simulink model "CM670A_HwAg1Meas"  (R2013b)
settings: Solver=FixedStepDiscrete  SolverMode=SingleTasking  StartTime=0.0  StopTime=22  FixedStep=0.002  RelTol=1e-3
values from neighbouring files (symbols this model uses):
  ELECGLBPRM_DEGPERREV_DEGPERREV_F32 = DataDict.Constant    [CM670A_HwAg1Meas_DataDict.m]
  ELECGLBPRM_HWAGCENTROFFS_HWDEG_F32 = DataDict.Constant    [CM670A_HwAg1Meas_DataDict.m]
  ELECGLBPRM_HWAGSATNLOWRLIM_HWDEG_F32 = DataDict.Constant    [CM670A_HwAg1Meas_DataDict.m]
  ELECGLBPRM_HWAGSATNUPPRLIM_HWDEG_F32 = DataDict.Constant    [CM670A_HwAg1Meas_DataDict.m]
  ELECGLBPRM_HWAGSCA_ULS_F32 = DataDict.Constant    [CM670A_HwAg1Meas_DataDict.m]
  ELECGLBPRM_HWAGSPURGEARRAT_ULS_F32 = DataDict.Constant    [CM670A_HwAg1Meas_DataDict.m]
  ELECGLBPRM_HWAGSPURTORINGGEARRATSNSR0_ULS_F32 = DataDict.Constant    [CM670A_HwAg1Meas_DataDict.m]
  ELECGLBPRM_HWAGSPURTORINGGEARRATSNSR1_ULS_F32 = DataDict.Constant    [CM670A_HwAg1Meas_DataDict.m]
  ELECGLBPRM_NOFLT_CNT_U08 = DataDict.Constant    [CM670A_HwAg1Meas_DataDict.m]
  ELECGLBPRM_OFFSTRIMNOTPRFMD_CNT_U08 = DataDict.Constant    [CM670A_HwAg1Meas_DataDict.m]
  ELECGLBPRM_PRTCLFLT_CNT_U08 = DataDict.Constant    [CM670A_HwAg1Meas_DataDict.m]
  ELECGLBPRM_SKIPSTEPFLT_CNT_U08 = DataDict.Constant    [CM670A_HwAg1Meas_DataDict.m]
  ELECGLBPRM_SNSRINTFLT_CNT_U08 = DataDict.Constant    [CM670A_HwAg1Meas_DataDict.m]
  ELECGLBPRM_VRNRERRFLT_CNT_U08 = DataDict.Constant    [CM670A_HwAg1Meas_DataDict.m]
  HWAG10THTOOTHTRIG_CNT_U08 = DataDict.ConfigParam    [CM670A_HwAg1Meas_DataDict.m]
  HWAG11THTOOTHTRIG_CNT_U08 = DataDict.ConfigParam    [CM670A_HwAg1Meas_DataDict.m]
  HwAg1IfFlt = DataDict.NTC    [CM670A_HwAg1Meas_DataDict.m]
  HwAg1MeasHwAg1IfFltFailStep = DataDict.Calibration    [CM670A_HwAg1Meas_DataDict.m]
  HwAg1MeasHwAg1IfFltPassStep = DataDict.Calibration    [CM670A_HwAg1Meas_DataDict.m]
  HwAg1MeasHwAg1Snsr0PrtclFltFailStep = DataDict.Calibration    [CM670A_HwAg1Meas_DataDict.m]
  HwAg1MeasHwAg1Snsr0PrtclFltPassStep = DataDict.Calibration    [CM670A_HwAg1Meas_DataDict.m]
  HwAg1MeasHwAg1Snsr1PrtclFltFailStep = DataDict.Calibration    [CM670A_HwAg1Meas_DataDict.m]
  HwAg1MeasHwAg1Snsr1PrtclFltPassStep = DataDict.Calibration    [CM670A_HwAg1Meas_DataDict.m]
  HwAg1MeasSnsr0Rev = DataDict.Calibration    [CM670A_HwAg1Meas_DataDict.m]
  HwAg1MeasSnsr1Rev = DataDict.Calibration    [CM670A_HwAg1Meas_DataDict.m]
  HwAg1MeasStep = DataDict.Calibration    [CM670A_HwAg1Meas_DataDict.m]
  HwAg1MeasVrnrErrThd = DataDict.Calibration    [CM670A_HwAg1Meas_DataDict.m]
  HwAg1MfgFlt = DataDict.NTC    [CM670A_HwAg1Meas_DataDict.m]
  HwAg1Snsr0PrtclFlt = DataDict.NTC    [CM670A_HwAg1Meas_DataDict.m]
  HwAg1Snsr1PrtclFlt = DataDict.NTC    [CM670A_HwAg1Meas_DataDict.m]
undefined symbols (not defined in the file or in its folder): NtcSts1, sigbuilder_block, SigQlfr1
libraries: simulink x30, NxtrNvM x3
(part 2 of 5)

== system CM670A_HwAg1Meas/HwAg1Meas/HwAg1MeasPer3 ==
  note: Follow below steps in same order:
      |
      | 1. Check the Sensor Seq Number
      |    1a. Check Sensor Seq Number Logic first
      |    1b. Execute RawHwAgRead
      |    1c. Clear RSENT2CSC = 2046U;
      |    1d. FRS Flag Check: If the RegInpRSENT2FRS==1,  Read the RegInpRSENT2FND
      |    1e. SYNCHRONIZATION PULSE Logic
      |
      | Design Note: Registers Read must be done once only. (Pl. see Design Rational Section for detail)
  RegInpRSENT2CS : Inport
  RegInpRSENT4FRXD : Inport  Port=2
  RegInpRSENT2NRS : Inport  Port=3
  RegInpRSENT2FRS : Inport  Port=4
  RegInpRSENT2FND : Inport  Port=5
  function : TriggerPort  TriggerType=function-call
  Constant : Constant  Value=HWAG11THTOOTHTRIG_CNT_U08
      settings: AttributesFormatString=%<Value>.EngVal = 2
  CopyRight2 : Subsystem  Description=|  mask(Copyright Information){none=on}
      | Copyright info block.                                               
      |                                                                     
      | Place copyright information at the top of every subsystem in design.
      mask prompts: none "No parameters"
      mask help: Place copyright information at the top of every subsystem in design.
      mask Display:
      | NxtrConf = 'Nexteer Confidential';
      | 
      | sys = bdroot; %handle for the current model ("system")
      | first = get_param(sys,'Created');
      | first = first(end-3:end);  %year is last four digits
      | 
      | last = get_param(sys,'LastModifiedDate');
      | if isempty(last)
      |     last = datestr(now,'yyyy');
      | else
      |     last = last(end-3:end);
      | end
      | 
      | if strcmp(first,last)
      |     fprintf('%s -- Copyright %s Nexteer',NxtrConf,first)
      | else
      |     fprintf('%s -- %s%s- %s Nexteer',NxtrConf,char(169),first,last)
      | end
  Data Store Read1 : DataStoreRead  DataStoreName=HwAg1SnsrTrigNr
  If1 : If  RequirementInfo={} %GIDa_01715eb0_255b_4dbd_b172_69669054b224  NumInputs=2  IfExpression=u1 == u2
  Merge : Merge
  Merge1 : Merge
  Snsr1Read : Subsystem  RequirementInfo={} %GIDa_dd29c1a1_900c_4b66_9138_b93d32baa948  TreatAsAtomicUnit=on
  Snsr1Read1 : Subsystem  RequirementInfo={} %GIDa_89898eab_9f67_4e64_9ea2_3164f9bb1266  TreatAsAtomicUnit=on
  HwAg1Snsr1Raw : Outport
  HwAg1Snsr1TestOk : Outport  Port=2
  wires:
  If1/2 -> Snsr1Read1/Action
  If1/1 -> Snsr1Read/Action
  Snsr1Read/1(HwAg1Snsr1Raw) -> Merge/1
  Snsr1Read1/2(HwAg1Snsr1TestOk) -> Merge1/2
  Snsr1Read/2(HwAg1Snsr1TestOk) -> Merge1/1
  Snsr1Read1/1(HwAg1Snsr1Raw) -> Merge/2
  RegInpRSENT2FRS/1 -> Snsr1Read/4(RegInpRSENT2FRS)
  RegInpRSENT2NRS/1 -> Snsr1Read/3(RegInpRSENT2NRS)
  RegInpRSENT4FRXD/1 -> Snsr1Read/2(RegInpRSENT4FRXD)
  RegInpRSENT2CS/1 -> Snsr1Read/1(RegInpRSENT2CS)
  RegInpRSENT2FND/1 -> Snsr1Read/5(RegInpRSENT2FND)
  Merge/1 -> HwAg1Snsr1Raw/1
  Merge1/1 -> HwAg1Snsr1TestOk/1
  Data Store Read1/1 -> If1/1
  Constant/1 -> If1/2

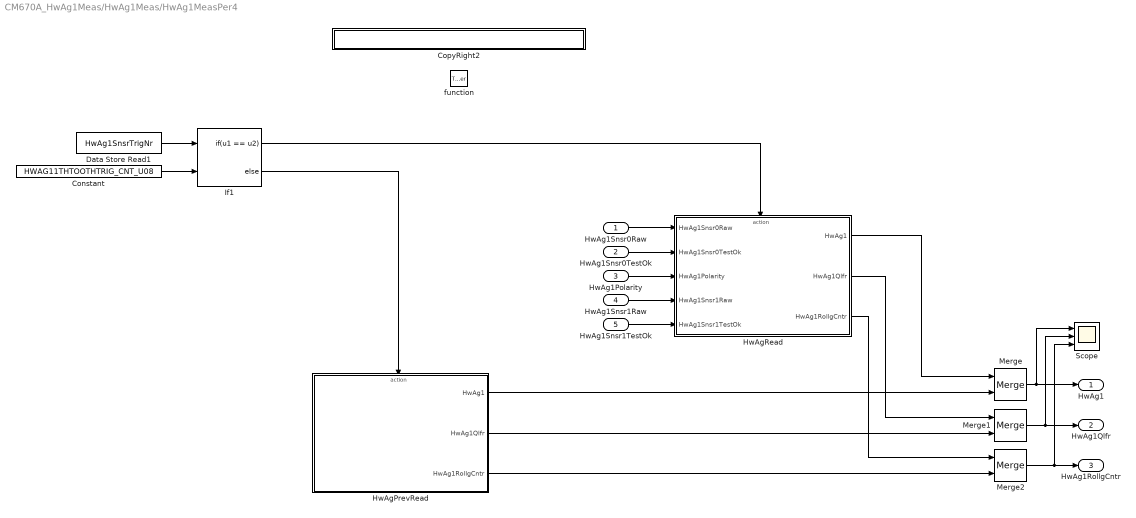
== system CM670A_HwAg1Meas/HwAg1Meas/HwAg1MeasPer4 ==
  HwAg1Snsr0Raw : Inport
  HwAg1Snsr0TestOk : Inport  Port=2
  HwAg1Polarity : Inport  Port=3
  HwAg1Snsr1Raw : Inport  Port=4
  HwAg1Snsr1TestOk : Inport  Port=5
  function : TriggerPort  TriggerType=function-call
  Constant : Constant  Value=HWAG11THTOOTHTRIG_CNT_U08
      settings: AttributesFormatString=%<Value>.EngVal = 2
  CopyRight2 : Subsystem  Description=|  mask(Copyright Information){none=on}
      | Copyright info block.                                               
      |                                                                     
      | Place copyright information at the top of every subsystem in design.
      mask prompts: none "No parameters"
      mask help: Place copyright information at the top of every subsystem in design.
      mask Display:
      | NxtrConf = 'Nexteer Confidential';
      | 
      | sys = bdroot; %handle for the current model ("system")
      | first = get_param(sys,'Created');
      | first = first(end-3:end);  %year is last four digits
      | 
      | last = get_param(sys,'LastModifiedDate');
      | if isempty(last)
      |     last = datestr(now,'yyyy');
      | else
      |     last = last(end-3:end);
      | end
      | 
      | if strcmp(first,last)
      |     fprintf('%s -- Copyright %s Nexteer',NxtrConf,first)
      | else
      |     fprintf('%s -- %s%s- %s Nexteer',NxtrConf,char(169),first,last)
      | end
  Data Store Read1 : DataStoreRead  DataStoreName=HwAg1SnsrTrigNr
  HwAgPrevRead : Subsystem  RequirementInfo={} %GIDa_7a5c75b0_c902_46a2_91c0_2fc119de8044  TreatAsAtomicUnit=on
  HwAgRead : Subsystem  RequirementInfo={} %GIDa_1616c0f0_8d95_4591_82f7_c51cd1b03528  TreatAsAtomicUnit=on
  If1 : If  RequirementInfo={} %GIDa_8cfb27f1_f362_4fee_af6b_0df0b8a33307  NumInputs=2  IfExpression=u1 == u2
  Merge : Merge
  Merge1 : Merge
  Merge2 : Merge
  Scope : Scope  NumInputPorts=3
      settings: TimeRange=22  YMin=-900~0~1  YMax=900~275~2  SaveName=ScopeData2
  HwAg1 : Outport  RequirementInfo={} %GIDa_6b698758_3f25_4f69_8482_aba696fb6d83
  HwAg1Qlfr : Outport  RequirementInfo={'linktype_rmi_doors' '0000cf45 (/ESG Group/FDD Module Requirements/EA4 Specific/CM690A_HwAg0Meas)' '#CM690A_30' 'true' 'REQ: CM690A_30' '' } %GIDa_a3b4fa17_774b_440f_aa44_3f1b92d803b2  Port=2
  HwAg1RollgCntr : Outport  RequirementInfo={'linktype_rmi_doors' '0000cf45 (/ESG Group/FDD Module Requirements/EA4 Specific/CM690A_HwAg0Meas)' '#CM690A_31' 'true' 'REQ: CM690A_31' '' } %GIDa_ac5eeb48_7c4b_45fd_afbe_ed47feb8fd90  Port=3
  wires:
  If1/2 -> HwAgPrevRead/Action
  If1/1 -> HwAgRead/Action
  Merge/1 -> Scope/1, HwAg1/1
  Merge1/1 -> Scope/2, HwAg1Qlfr/1
  Merge2/1 -> Scope/3, HwAg1RollgCntr/1
  HwAgRead/1(HwAg1) -> Merge/1
  HwAgRead/2(HwAg1Qlfr) -> Merge1/1
  HwAgRead/3(HwAg1RollgCntr) -> Merge2/1
  HwAgPrevRead/1(HwAg1) -> Merge/2
  HwAgPrevRead/2(HwAg1Qlfr) -> Merge1/2
  HwAgPrevRead/3(HwAg1RollgCntr) -> Merge2/2
  HwAg1Snsr1Raw/1 -> HwAgRead/4(HwAg1Snsr1Raw)
  HwAg1Snsr0TestOk/1 -> HwAgRead/2(HwAg1Snsr0TestOk)
  HwAg1Snsr0Raw/1 -> HwAgRead/1(HwAg1Snsr0Raw)
  HwAg1Snsr1TestOk/1 -> HwAgRead/5(HwAg1Snsr1TestOk)
  HwAg1Polarity/1 -> HwAgRead/3(HwAg1Polarity)
  Data Store Read1/1 -> If1/1
  Constant/1 -> If1/2

== system CM670A_HwAg1Meas/HwAg1Meas/HwAg1MeasPer5 ==
  note: Information Only:
      | - Trim not performed Ntc
  function : TriggerPort  TriggerType=function-call
  Constant : Constant  Value=HwAg1MfgFlt
  CopyRight2 : Subsystem  Description=|  mask(Copyright Information){none=on}
      | Copyright info block.                                               
      |                                                                     
      | Place copyright information at the top of every subsystem in design.
      mask prompts: none "No parameters"
      mask help: Place copyright information at the top of every subsystem in design.
      mask Display:
      | NxtrConf = 'Nexteer Confidential';
      | 
      | sys = bdroot; %handle for the current model ("system")
      | first = get_param(sys,'Created');
      | first = first(end-3:end);  %year is last four digits
      | 
      | last = get_param(sys,'LastModifiedDate');
      | if isempty(last)
      |     last = datestr(now,'yyyy');
      | else
      |     last = last(end-3:end);
      | end
      | 
      | if strcmp(first,last)
      |     fprintf('%s -- Copyright %s Nexteer',NxtrConf,first)
      | else
      |     fprintf('%s -- %s%s- %s Nexteer',NxtrConf,char(169),first,last)
      | end
  Data Store Read1 : DataStoreRead  DataStoreName=HwAg1OffsTrimPrfmdSts
  Ground : Ground
  If : If  IfExpression=(u1 ~= 0)
  If Action Subsystem : Subsystem  RequirementInfo={'linktype_rmi_doors' '0000cf44 (/ESG Group/FDD Module Requirements/EA4 Specific/CM670A_HwAg1Meas)' '#CM670A_84' 'true' 'REQ: CM670A_84' '' } %GIDa_93c0c2f6_38ee_4160_b051_f0ab663f9dc9  TreatAsAtomicUnit=on
  If Action Subsystem1 : Subsystem  RequirementInfo={'linktype_rmi_doors' '0000cf44 (/ESG Group/FDD Module Requirements/EA4 Specific/CM670A_HwAg1Meas)' '#CM670A_82' 'true' 'REQ: CM670A_82' '' } %GIDa_fa6d762f_0a06_4ac8_8aec_4f8d74e26f90  TreatAsAtomicUnit=on
  Merge : Merge
  Merge1 : Merge
  Scope : Scope  NumInputPorts=2
      settings: YMin=-5~-5  YMax=5~5  SaveName=ScopeData3
  SetNtcSts : Subsystem  RequirementInfo={'linktype_rmi_doors' '0000cf44 (/ESG Group/FDD Module Requirements/EA4 Specific/CM670A_HwAg1Meas)' '#CM670A_78' 'true' 'REQ: CM670A_78' '' } %GIDa_9e3edb63_7888_44cf_a718_771f9129b5ad
  wires:
  Ground/1 -> SetNtcSts/4(DebStep)
  Constant/1 -> SetNtcSts/1(NtcNr)
  Data Store Read1/1 -> If/1
  If/1 -> If Action Subsystem/Action
  If/2 -> If Action Subsystem1/Action
  If Action Subsystem/1(ParamByte) -> Merge/1
  If Action Subsystem1/1(ParamByte) -> Merge/2
  If Action Subsystem/2(TestOk) -> Merge1/1
  If Action Subsystem1/2(TestOk) -> Merge1/2
  Merge/1 -> Scope/1, SetNtcSts/2(NtcStInfo)  "ParamByte"
  Merge1/1 -> Scope/2, SetNtcSts/3(NtcSts)  "TestOk"

== system CM670A_HwAg1Meas/Simulated_Input/CopyRight2 ==

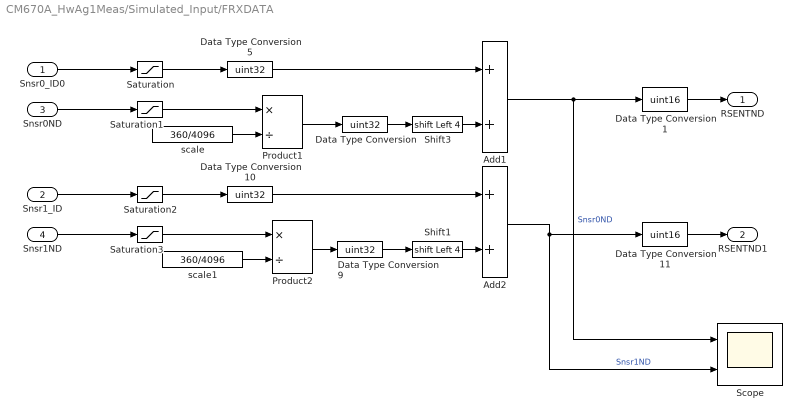
== system CM670A_HwAg1Meas/Simulated_Input/FRXDATA ==
  Snsr0_ID0 : Inport
  Snsr1_ID : Inport  Port=2
  Snsr0ND : Inport  Port=3
  Snsr1ND : Inport  Port=4
  Add1 : Sum
  Add2 : Sum
  Data Type Conversion : DataTypeConversion  OutDataTypeStr=uint32
  Data Type Conversion1 : DataTypeConversion  OutDataTypeStr=uint16
  Data Type Conversion10 : DataTypeConversion  OutDataTypeStr=uint32  SaturateOnIntegerOverflow=on
  Data Type Conversion11 : DataTypeConversion  OutDataTypeStr=uint16
  Data Type Conversion5 : DataTypeConversion  OutDataTypeStr=uint32
  Data Type Conversion9 : DataTypeConversion  OutDataTypeStr=uint32
  Product1 : Product  Inputs=*/
  Product2 : Product  Inputs=*/
  Saturation : Saturate  UpperLimit=1  LowerLimit=0
  Saturation1 : Saturate  UpperLimit=360  LowerLimit=0
  Saturation2 : Saturate  UpperLimit=1  LowerLimit=0
  Saturation3 : Saturate  UpperLimit=360  LowerLimit=0
  Scope : Scope  NumInputPorts=2
      settings: YMin=1.02005e+09~0  YMax=1.12743e+09~6e+08
  Shift1 : ArithShift  BitShiftNumber=4  BitShiftDirection=Left
  Shift3 : ArithShift  BitShiftNumber=4  BitShiftDirection=Left
  scale : Constant  Value=360/4096
  scale1 : Constant  Value=360/4096
  RSENTND : Outport
  RSENTND1 : Outport  Port=2
  wires:
  Snsr0ND/1 -> Saturation1/1
  scale/1 -> Product1/2
  Product1/1 -> Data Type Conversion/1
  Data Type Conversion1/1 -> RSENTND/1
  Snsr0_ID0/1 -> Saturation/1
  Data Type Conversion5/1 -> Add1/1
  Data Type Conversion/1 -> Shift3/1
  Add1/1 -> Scope/1, Data Type Conversion1/1  "Snsr0ND"
  Snsr1ND/1 -> Saturation3/1
  scale1/1 -> Product2/2
  Product2/1 -> Data Type Conversion9/1
  Snsr1_ID/1 -> Saturation2/1
  Data Type Conversion10/1 -> Add2/1
  Data Type Conversion9/1 -> Shift1/1
  Data Type Conversion11/1 -> RSENTND1/1
  Add2/1 -> Data Type Conversion11/1, Scope/2  "Snsr1ND"
  Saturation/1 -> Data Type Conversion5/1
  Saturation1/1 -> Product1/1
  Saturation2/1 -> Data Type Conversion10/1
  Saturation3/1 -> Product2/1
  Shift3/1 -> Add1/2
  Shift1/1 -> Add2/2

== system CM670A_HwAg1Meas/Simulated_Input/FRXDATA1 ==
  Snsr0_CS : Inport
  Snsr1_CS : Inport  Port=2
  Snsr0_FRS : Inport  Port=3
  Snsr1_FRS : Inport  Port=4
  Add1 : Sum
  Add2 : Sum
  Data Type Conversion{,1,5,9,11} (5 alike) : DataTypeConversion  OutDataTypeStr=uint32
  Data Type Conversion10 : DataTypeConversion  OutDataTypeStr=uint32  SaturateOnIntegerOverflow=on
  Scope : Scope  NumInputPorts=2
      settings: YMin=1.02005e+09~0  YMax=1.12743e+09~6e+08
  Shift1 : ArithShift  BitShiftNumber=1  BitShiftDirection=Left
  Shift3 : ArithShift  BitShiftNumber=1  BitShiftDirection=Left
  Snsr0CS : Outport
  Snsr1CS : Outport  Port=2
  wires:
  Data Type Conversion9/1 -> Add2/2
  Data Type Conversion/1 -> Add1/2
  Snsr1_CS/1 -> Data Type Conversion10/1
  Snsr0_CS/1 -> Data Type Conversion5/1
  Add2/1 -> Scope/2, Data Type Conversion11/1  "Snsr1ND"
  Data Type Conversion11/1 -> Snsr1CS/1
  Data Type Conversion10/1 -> Shift1/1
  Add1/1 -> Data Type Conversion1/1, Scope/1  "Snsr0ND"
  Data Type Conversion5/1 -> Shift3/1
  Data Type Conversion1/1 -> Snsr0CS/1
  Snsr0_FRS/1 -> Data Type Conversion/1
  Snsr1_FRS/1 -> Data Type Conversion9/1
  Shift3/1 -> Add1/1
  Shift1/1 -> Add2/1

== system CM670A_HwAg1Meas/Simulated_Input/FRXDATA2 ==
  Snsr0_FCCN : Inport
  Snsr1_FCCN : Inport  Port=2
  Snsr0_Data : Inport  Port=3
  Snsr1_Data : Inport  Port=4
  Add1 : Sum
  Add2 : Sum
  Data Type Conversion{,1,5,9,11} (5 alike) : DataTypeConversion  OutDataTypeStr=uint32
  Data Type Conversion10 : DataTypeConversion  OutDataTypeStr=uint32  SaturateOnIntegerOverflow=on
  Scope : Scope  NumInputPorts=2
      settings: YMin=1.02005e+09~0  YMax=1.12743e+09~6e+08
  Shift1 : ArithShift  BitShiftNumber=28  BitShiftDirection=Left
  Shift3 : ArithShift  BitShiftNumber=28  BitShiftDirection=Left
  Snsr0FRXD : Outport
  Snsr1FRXD : Outport  Port=2
  wires:
  Shift1/1 -> Add2/1
  Shift3/1 -> Add1/1
  Snsr1_Data/1 -> Data Type Conversion9/1
  Snsr0_Data/1 -> Data Type Conversion/1
  Data Type Conversion1/1 -> Snsr0FRXD/1
  Data Type Conversion5/1 -> Shift3/1
  Add1/1 -> Scope/1, Data Type Conversion1/1  "Snsr0ND"
  Data Type Conversion10/1 -> Shift1/1
  Data Type Conversion11/1 -> Snsr1FRXD/1
  Add2/1 -> Data Type Conversion11/1, Scope/2  "Snsr1ND"
  Snsr0_FCCN/1 -> Data Type Conversion5/1
  Snsr1_FCCN/1 -> Data Type Conversion10/1
  Data Type Conversion/1 -> Add1/2
  Data Type Conversion9/1 -> Add2/2

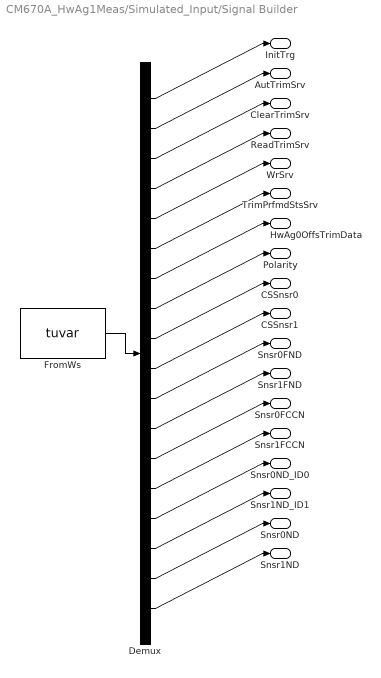
== system CM670A_HwAg1Meas/Simulated_Input/Signal Builder ==
  Demux : Demux  Tag=STV Demux  Outputs=18
  FromWs : FromWorkspace  Tag=STV FromWs  VariableName=tuvar  SampleTime=0  OutputAfterFinalValue=Holding final value
      SigBuilderData=|
      | common.afterFinalStr = 'Hold final value'
      | common.sampleTime = '0'
      | dataSet(1).timeRange = [0 22]
      | dataSet(1).name = 'IdealSignal'
      | dataSet(2).timeRange = [0 22]
      | dataSet(2).name = 'Faults'
      | dataSet(3).timeRange = [0 22]
      | dataSet(3).name = 'Service'
      | dataSet(4).timeRange = [0 22]
      | dataSet(4).name = 'RollOver'
      | sbobj.Groups(1).Name = 'IdealSignal'
      | sbobj.Groups(1).Signals(1).Name = 'InitTrg'
      | sbobj.Groups(1).Signals(1).XData = [0 0.02 0.02 0.06 0.06 22]
      | sbobj.Groups(1).Signals(1).YData = [0 0 1 1 0 0]
      | sbobj.Groups(1).Signals(2).Name = 'AutTrimSrv'
      | sbobj.Groups(1).Signals(2).XData = [0 22]
      | sbobj.Groups(1).Signals(2).YData = [0 0]
      | sbobj.Groups(1).Signals(3).Name = 'ClearTrimSrv'
      | sbobj.Groups(1).Signals(3).XData = [0 22]
      | sbobj.Groups(1).Signals(3).YData = [0 0]
      | sbobj.Groups(1).Signals(4).Name = 'ReadTrimSrv'
      | sbobj.Groups(1).Signals(4).XData = [0 22]
      | sbobj.Groups(1).Signals(4).YData = [0 0]
      | sbobj.Groups(1).Signals(5).Name = 'WrSrv'
      | sbobj.Groups(1).Signals(5).XData = [0 0.04 0.04 0.08 0.08 22]
      | sbobj.Groups(1).Signals(5).YData = [0 0 1 1 0 0]
      | sbobj.Groups(1).Signals(6).Name = 'TrimPrfmdStsSrv'
      | sbobj.Groups(1).Signals(6).XData = [0 22]
      | sbobj.Groups(1).Signals(6).YData = [0 0]
      | sbobj.Groups(1).Signals(7).Name = 'HwAg0OffsTrimData'
      | sbobj.Groups(1).Signals(7).XData = [0 22]
      | sbobj.Groups(1).Signals(7).YData = [0 0]
      | sbobj.Groups(1).Signals(8).Name = 'Polarity'
      | sbobj.Groups(1).Signals(8).XData = [0 22]
      | sbobj.Groups(1).Signals(8).YData = [1 1]
      | sbobj.Groups(1).Signals(9).Name = 'CSSnsr0'
      | sbobj.Groups(1).Signals(9).XData = [0 22]
      | sbobj.Groups(1).Signals(9).YData = [0 0]
      | sbobj.Groups(1).Signals(10).Name = 'CSSnsr1'
      | sbobj.Groups(1).Signals(10).XData = [0 22]
      | sbobj.Groups(1).Signals(10).YData = [0 0]
      | sbobj.Groups(1).Signals(11).Name = 'Snsr0FND'
      | sbobj.Groups(1).Signals(11).XData = [0 22]
      | sbobj.Groups(1).Signals(11).YData = [1 1]
      | sbobj.Groups(1).Signals(12).Name = 'Snsr1FND'
      | sbobj.Groups(1).Signals(12).XData = [0 22]
      | sbobj.Groups(1).Signals(12).YData = [1 1]
      | sbobj.Groups(1).Signals(13).Name = 'Snsr0FCCN'
      | sbobj.Groups(1).Signals(13).XData = [0 22]
      | sbobj.Groups(1).Signals(13).YData = [0 0]
      | sbobj.Groups(1).Signals(14).Name = 'Snsr1FCCN'
      | sbobj.Groups(1).Signals(14).XData = [0 22]
      | sbobj.Groups(1).Signals(14).YData = [0 0]
      | sbobj.Groups(1).Signals(15).Name = 'Snsr0ND_ID0'
      | sbobj.Groups(1).Signals(15).XData = [0 22]
      | sbobj.Groups(1).Signals(15).YData = [0 0]
      | sbobj.Groups(1).Signals(16).Name = 'Snsr1ND_ID1'
      | sbobj.Groups(1).Signals(16).XData = [0 22]
      | sbobj.Groups(1).Signals(16).YData = [1 1]
      | sbobj.Groups(1).Signals(17).Name = 'Snsr0ND'
      | sbobj.Groups(1).Signals(17).XData = [0 2 2 4 4 6 6 8 8 10 10 12 12 14 14 16 16 18 18 20 20 22]
      | sbobj.Groups(1).Signals(17).YData = [0 359.9 0 359.9 0 359.9 0 359.9 0 359.9 0 359.9 0 359.9 0 359.9 0 359.9 0 359.9 0 359.9]
      | sbobj.Groups(1).Signals(18).Name = 'Snsr1ND'
      | sbobj.Groups(1).Signals(18).XData = [0 2.2000022 2.2000022 4.4000044 4.4000044 6.60000660001 6.60000660001 8.80000880001 8.80000880001 11.000011 11.000011 13.2000132 13.2000132 15.4000154 15.4000154 17.6000176 17.6000176 19.8000198 19.8000198 22]
      | sbobj.Groups(1).Signals(18).YData = [0 359.9 0 359.9 0 359.9 0 359.9 0 359.9 0 359.9 0 359.9 0 359.9 0 359.9 0 359.896401]
      | sbobj.Groups(1).TimeRange = [0 22]
      | sbobj.Groups(2).Name = 'Faults'
      | sbobj.Groups(2).Signals(1).Name = 'InitTrg'
      | sbobj.Groups(2).Signals(1).XData = [0 0.02 0.02 0.06 0.06 22]
      | sbobj.Groups(2).Signals(1).YData = [0 0 1 1 0 0]
      | sbobj.Groups(2).Signals(2).Name = 'AutTrimSrv'
      | sbobj.Groups(2).Signals(2).XData = [0 22]
      | sbobj.Groups(2).Signals(2).YData = [0 0]
      | sbobj.Groups(2).Signals(3).Name = 'ClearTrimSrv'
      | sbobj.Groups(2).Signals(3).XData = [0 22]
      | sbobj.Groups(2).Signals(3).YData = [0 0]
      | sbobj.Groups(2).Signals(4).Name = 'ReadTrimSrv'
      | sbobj.Groups(2).Signals(4).XData = [0 22]
      | sbobj.Groups(2).Signals(4).YData = [0 0]
      | sbobj.Groups(2).Signals(5).Name = 'WrSrv'
      | sbobj.Groups(2).Signals(5).XData = [0 0.06 0.06 0.12 0.12 22]
      | sbobj.Groups(2).Signals(5).YData = [0 0 1 1 0 0]
      | sbobj.Groups(2).Signals(6).Name = 'TrimPrfmdStsSrv'
      | sbobj.Groups(2).Signals(6).XData = [0 22]
      | sbobj.Groups(2).Signals(6).YData = [0 0]
      | sbobj.Groups(2).Signals(7).Name = 'HwAg0OffsTrimData'
      | sbobj.Groups(2).Signals(7).XData = [0 22]
      | sbobj.Groups(2).Signals(7).YData = [0 0]
      | sbobj.Groups(2).Signals(8).Name = 'Polarity'
      | sbobj.Groups(2).Signals(8).XData = [0 11 11 22]
      | sbobj.Groups(2).Signals(8).YData = [-1 -1 1 1]
      | sbobj.Groups(2).Signals(9).Name = 'CSSnsr0'
      | sbobj.Groups(2).Signals(9).XData = [0 2.54 2.54 2.88 2.88 22]
      | sbobj.Groups(2).Signals(9).YData = [0 0 2 2 0 0]
      | sbobj.Groups(2).Signals(10).Name = 'CSSnsr1'
      | sbobj.Groups(2).Signals(10).XData = [0 4.36 4.36 4.78 4.78 22]
      | sbobj.Groups(2).Signals(10).YData = [0 0 2 2 0 0]
      | sbobj.Groups(2).Signals(11).Name = 'Snsr0FND'
      | sbobj.Groups(2).Signals(11).XData = [0 14.54 14.54 14.78 14.78 22]
      | sbobj.Groups(2).Signals(11).YData = [1 1 0 0 1 1]
      | sbobj.Groups(2).Signals(12).Name = 'Snsr1FND'
      | sbobj.Groups(2).Signals(12).XData = [0 15.66 15.66 15.94 15.94 22]
      | sbobj.Groups(2).Signals(12).YData = [1 1 0 0 1 1]
      | sbobj.Groups(2).Signals(13).Name = 'Snsr0FCCN'
      | sbobj.Groups(2).Signals(13).XData = [0 12.02 12.02 12.26 12.26 22]
      | sbobj.Groups(2).Signals(13).YData = [0 0 1 1 0 0]
      | sbobj.Groups(2).Signals(14).Name = 'Snsr1FCCN'
      | sbobj.Groups(2).Signals(14).XData = [0 12.92 12.92 13.2 13.2 22]
      | sbobj.Groups(2).Signals(14).YData = [0 0 2 2 0 0]
      | sbobj.Groups(2).Signals(15).Name = 'Snsr0ND_ID0'
      | sbobj.Groups(2).Signals(15).XData = [0 6.46 6.46 6.8 6.8 22]
      | sbobj.Groups(2).Signals(15).YData = [0 0 1 1 0 0]
      | sbobj.Groups(2).Signals(16).Name = 'Snsr1ND_ID1'
      | sbobj.Groups(2).Signals(16).XData = [0 8.8 8.8 9.32 9.32 22]
      | sbobj.Groups(2).Signals(16).YData = [1 1 0 0 1 1]
      | sbobj.Groups(2).Signals(17).Name = 'Snsr0ND'
      | sbobj.Groups(2).Signals(17).XData = [0 2 2 4 4 6 6 8 8 10 10 12 12 14 14 16 16 18 18 20 20 22]
      | sbobj.Groups(2).Signals(17).YData = [0 359.9 0 359.9 0 359.9 0 359.9 0 359.9 0 359.9 0 359.9 0 359.9 0 359.9 0 359.9 0 350]
      | sbobj.Groups(2).Signals(18).Name = 'Snsr1ND'
      | sbobj.Groups(2).Signals(18).XData = [0 2.2000022 2.2000022 4.4000044 4.4000044 6.60000660001 6.60000660001 8.80000880001 8.80000880001 11.000011 11.000011 13.2000132 13.2000132 15.4000154 15.4000154 17.6000176 17.6000176 20 20 22]
      | sbobj.Groups(2).Signals(18).YData = [0 359.9 0 359.9 0 359.9 0 359.9 0 359.9 0 359.9 0 359.9 0 359.9 0 359.9 0 350]
      | sbobj.Groups(2).TimeRange = [0 22]
      | sbobj.Groups(3).Name = 'Service'
      | sbobj.Groups(3).Signals(1).Name = 'InitTrg'
      | sbobj.Groups(3).Signals(1).XData = [0 0.02 0.02 0.06 0.06 22]
      | sbobj.Groups(3).Signals(1).YData = [0 0 1 1 0 0]
      | sbobj.Groups(3).Signals(2).Name = 'AutTrimSrv'
      | sbobj.Groups(3).Signals(2).XData = [0 0.58 0.58 0.68 0.68 16 16 16.1 16.1 22]
      | sbobj.Groups(3).Signals(2).YData = [0 0 1 1 0 0 1 1 0 0]
      | sbobj.Groups(3).Signals(3).Name = 'ClearTrimSrv'
      | sbobj.Groups(3).Signals(3).XData = [0 0.34 4.1 4.1 4.16 4.16 9.98 9.98 10.06 10.06 22]
      | sbobj.Groups(3).Signals(3).YData = [0 0 0 1 1 0 0 1 1 0 0]
      | sbobj.Groups(3).Signals(4).Name = 'ReadTrimSrv'
      | sbobj.Groups(3).Signals(4).XData = [0 1.24 1.24 1.32 1.32 4.62 4.62 4.7 4.7 6.84 6.84 6.92 6.92 10.38 10.38 10.46 10.46 16.72 16.72 16.8 16.8 22]
      | sbobj.Groups(3).Signals(4).YData = [0 0 1 1 0 0 1 1 0 0 1 1 0 0 1 1 0 0 1 1 0 0]
      | sbobj.Groups(3).Signals(5).Name = 'WrSrv'
      | sbobj.Groups(3).Signals(5).XData = [0 6.22 6.22 6.3 6.3 22]
      | sbobj.Groups(3).Signals(5).YData = [0 0 1 1 0 0]
      | sbobj.Groups(3).Signals(6).Name = 'TrimPrfmdStsSrv'
      | sbobj.Groups(3).Signals(6).XData = [0 1.24 1.24 1.32 1.32 4.64 4.64 4.7 4.7 6.84 6.84 6.92 6.92 10.64 10.64 10.72 10.72 16.74 16.74 16.82 16.82 22]
      | sbobj.Groups(3).Signals(6).YData = [0 0 1 1 0 0 1 1 0 0 1 1 0 0 1 1 0 0 1 1 0 0]
      | sbobj.Groups(3).Signals(7).Name = 'HwAg0OffsTrimData'
      | sbobj.Groups(3).Signals(7).XData = [0 0.4 5.4 5.4 11.16 11.16 22]
      | sbobj.Groups(3).Signals(7).YData = [0 0 0 300 300 0 0]
      | sbobj.Groups(3).Signals(8).Name = 'Polarity'
      | sbobj.Groups(3).Signals(8).XData = [0 22]
      | sbobj.Groups(3).Signals(8).YData = [1 1]
      | sbobj.Groups(3).Signals(9).Name = 'CSSnsr0'
      | sbobj.Groups(3).Signals(9).XData = [0 22]
      | sbobj.Groups(3).Signals(9).YData = [0 0]
      | sbobj.Groups(3).Signals(10).Name = 'CSSnsr1'
      | sbobj.Groups(3).Signals(10).XData = [0 22]
      | sbobj.Groups(3).Signals(10).YData = [0 0]
      | sbobj.Groups(3).Signals(11).Name = 'Snsr0FND'
      | sbobj.Groups(3).Signals(11).XData = [0 22]
      | sbobj.Groups(3).Signals(11).YData = [1 1]
      | sbobj.Groups(3).Signals(12).Name = 'Snsr1FND'
      | sbobj.Groups(3).Signals(12).XData = [0 22]
      | sbobj.Groups(3).Signals(12).YData = [1 1]
      | sbobj.Groups(3).Signals(13).Name = 'Snsr0FCCN'
      | sbobj.Groups(3).Signals(13).XData = [0 22]
      | sbobj.Groups(3).Signals(13).YData = [0 0]
      | sbobj.Groups(3).Signals(14).Name = 'Snsr1FCCN'
      | sbobj.Groups(3).Signals(14).XData = [0 22]
      | sbobj.Groups(3).Signals(14).YData = [0 0]
      | sbobj.Groups(3).Signals(15).Name = 'Snsr0ND_ID0'
      | sbobj.Groups(3).Signals(15).XData = [0 22]
      | sbobj.Groups(3).Signals(15).YData = [0 0]
      | sbobj.Groups(3).Signals(16).Name = 'Snsr1ND_ID1'
      | sbobj.Groups(3).Signals(16).XData = [0 22]
      | sbobj.Groups(3).Signals(16).YData = [1 1]
      | sbobj.Groups(3).Signals(17).Name = 'Snsr0ND'
      | sbobj.Groups(3).Signals(17).XData = [0 2 2 4 4 6 6 8 8 10 10 12 12 14 14 16 16 18 18 20 20 22]
      | sbobj.Groups(3).Signals(17).YData = [0 359.9 0 359.9 0 359.9 0 359.9 0 359.9 0 359.9 0 359.9 0 359.9 0 359.9 0 359.9 0 359.9]
      | sbobj.Groups(3).Signals(18).Name = 'Snsr1ND'
      | sbobj.Groups(3).Signals(18).XData = [0 2.2000022 2.2000022 4.4000044 4.4000044 6.60000660001 6.60000660001 8.80000880001 8.80000880001 11.000011 11.000011 13.2000132 13.2000132 15.4000154 15.4000154 17.6000176 17.6000176 19.8000198 19.8000198 22]
      | sbobj.Groups(3).Signals(18).YData = [0 359.9 0 359.9 0 359.9 0 359.9 0 359.9 0 359.9 0 359.9 0 359.9 0 359.9 0 359.896401]
      | sbobj.Groups(3).TimeRange = [0 22]
      | sbobj.Groups(4).Name = 'RollOver'
      | sbobj.Groups(4).Signals(1).Name = 'InitTrg'
      | sbobj.Groups(4).Signals(1).XData = [0 0.02 0.02 0.06 0.06 22]
      | sbobj.Groups(4).Signals(1).YData = [0 0 1 1 0 0]
      | sbobj.Groups(4).Signals(2).Name = 'AutTrimSrv'
      | sbobj.Groups(4).Signals(2).XData = [0 0.58 0.58 0.68 0.68 15.76 16.1 22]
      | sbobj.Groups(4).Signals(2).YData = [0 0 1 1 0 0 0 0]
      | sbobj.Groups(4).Signals(3).Name = 'ClearTrimSrv'
      | sbobj.Groups(4).Signals(3).XData = [0 22]
      | sbobj.Groups(4).Signals(3).YData = [0 0]
      | sbobj.Groups(4).Signals(4).Name = 'ReadTrimSrv'
      | sbobj.Groups(4).Signals(4).XData = [0 1.24 1.24 1.32 1.32 4.62 4.62 4.7 4.7 6.84 6.84 6.92 6.92 10.38 10.38 10.46 10.46 16.72 16.72 16.8 16.8 22]
      | sbobj.Groups(4).Signals(4).YData = [0 0 1 1 0 0 1 1 0 0 1 1 0 0 1 1 0 0 1 1 0 0]
      | sbobj.Groups(4).Signals(5).Name = 'WrSrv'
      | sbobj.Groups(4).Signals(5).XData = [0 22]
      | sbobj.Groups(4).Signals(5).YData = [0 0]
      | sbobj.Groups(4).Signals(6).Name = 'TrimPrfmdStsSrv'
      | sbobj.Groups(4).Signals(6).XData = [0 1.24 1.24 1.32 1.32 4.64 4.64 4.7 4.7 6.84 6.84 6.92 6.92 10.64 10.64 10.72 10.72 16.74 16.74 16.82 16.82 22]
      | sbobj.Groups(4).Signals(6).YData = [0 0 1 1 0 0 1 1 0 0 1 1 0 0 1 1 0 0 1 1 0 0]
      | sbobj.Groups(4).Signals(7).Name = 'HwAg0OffsTrimData'
      | sbobj.Groups(4).Signals(7).XData = [0 0.4 5.4 5.4 11.16 11.16 22]
      | sbobj.Groups(4).Signals(7).YData = [0 0 0 300 300 0 0]
      | sbobj.Groups(4).Signals(8).Name = 'Polarity'
      | sbobj.Groups(4).Signals(8).XData = [0 22]
      | sbobj.Groups(4).Signals(8).YData = [1 1]
      | sbobj.Groups(4).Signals(9).Name = 'CSSnsr0'
      | sbobj.Groups(4).Signals(9).XData = [0 22]
      | sbobj.Groups(4).Signals(9).YData = [0 0]
      | sbobj.Groups(4).Signals(10).Name = 'CSSnsr1'
      | sbobj.Groups(4).Signals(10).XData = [0 22]
      | sbobj.Groups(4).Signals(10).YData = [0 0]
      | sbobj.Groups(4).Signals(11).Name = 'Snsr0FND'
      | sbobj.Groups(4).Signals(11).XData = [0 22]
      | sbobj.Groups(4).Signals(11).YData = [1 1]
      | sbobj.Groups(4).Signals(12).Name = 'Snsr1FND'
      | sbobj.Groups(4).Signals(12).XData = [0 22]
      | sbobj.Groups(4).Signals(12).YData = [1 1]
      | sbobj.Groups(4).Signals(13).Name = 'Snsr0FCCN'
      | sbobj.Groups(4).Signals(13).XData = [0 22]
      | sbobj.Groups(4).Signals(13).YData = [0 0]
      | sbobj.Groups(4).Signals(14).Name = 'Snsr1FCCN'
      | sbobj.Groups(4).Signals(14).XData = [0 22]
      | sbobj.Groups(4).Signals(14).YData = [0 0]
      | sbobj.Groups(4).Signals(15).Name = 'Snsr0ND_ID0'
      | sbobj.Groups(4).Signals(15).XData = [0 22]
      | sbobj.Groups(4).Signals(15).YData = [0 0]
      | sbobj.Groups(4).Signals(16).Name = 'Snsr1ND_ID1'
      | sbobj.Groups(4).Signals(16).XData = [0 22]
      | sbobj.Groups(4).Signals(16).YData = [1 1]
      | sbobj.Groups(4).Signals(17).Name = 'Snsr0ND'
      | sbobj.Groups(4).Signals(17).XData = [0 2 2 4 4 6 6 8 8 10 10 12 12 14 14 16 16 18 18 20 20 22]
      | sbobj.Groups(4).Signals(17).YData = [0 359.9 0 359.9 0 359.9 0 359.9 0 359.9 0 359.9 0 359.9 0 359.9 0 359.9 0 359.9 0 359.9]
      | sbobj.Groups(4).Signals(18).Name = 'Snsr1ND'
      | sbobj.Groups(4).Signals(18).XData = [0 2.2000022 2.2000022 4.4000044 4.4000044 6.60000660001 6.60000660001 8.80000880001 8.80000880001 11.000011 11.000011 13.2000132 13.2000132 15.4000154 15.4000154 17.6000176 17.6000176 19.8000198 19.8000198 22]
      | sbobj.Groups(4).Signals(18).YData = [0 359.9 0 359.9 0 359.9 0 359.9 0 359.9 0 359.9 0 359.9 0 359.9 0 359.9 0 359.896401]
      | sbobj.Groups(4).TimeRange = [0 22]
  InitTrg : Outport  Tag=STV Outport
  AutTrimSrv : Outport  Tag=STV Outport  Port=2
  ClearTrimSrv : Outport  Tag=STV Outport  Port=3
  ReadTrimSrv : Outport  Tag=STV Outport  Port=4
  WrSrv : Outport  Tag=STV Outport  Port=5
  TrimPrfmdStsSrv : Outport  Tag=STV Outport  Port=6
  HwAg0OffsTrimData : Outport  Tag=STV Outport  Port=7
  Polarity : Outport  Tag=STV Outport  Port=8
  CSSnsr0 : Outport  Tag=STV Outport  Port=9
  CSSnsr1 : Outport  Tag=STV Outport  Port=10
  Snsr0FND : Outport  Tag=STV Outport  Port=11
  Snsr1FND : Outport  Tag=STV Outport  Port=12
  Snsr0FCCN : Outport  Tag=STV Outport  Port=13
  Snsr1FCCN : Outport  Tag=STV Outport  Port=14
  Snsr0ND_ID0 : Outport  Tag=STV Outport  Port=15
  Snsr1ND_ID1 : Outport  Tag=STV Outport  Port=16
  Snsr0ND : Outport  Tag=STV Outport  Port=17
  Snsr1ND : Outport  Tag=STV Outport  Port=18
  wires:
  FromWs/1 -> Demux/1
  Demux/1 -> InitTrg/1
  Demux/2 -> AutTrimSrv/1
  Demux/3 -> ClearTrimSrv/1
  Demux/4 -> ReadTrimSrv/1
  Demux/5 -> WrSrv/1
  Demux/6 -> TrimPrfmdStsSrv/1
  Demux/7 -> HwAg0OffsTrimData/1
  Demux/8 -> Polarity/1
  Demux/9 -> CSSnsr0/1
  Demux/10 -> CSSnsr1/1
  Demux/11 -> Snsr0FND/1
  Demux/12 -> Snsr1FND/1
  Demux/13 -> Snsr0FCCN/1
  Demux/14 -> Snsr1FCCN/1
  Demux/15 -> Snsr0ND_ID0/1
  Demux/16 -> Snsr1ND_ID1/1
  Demux/17 -> Snsr0ND/1
  Demux/18 -> Snsr1ND/1

== system CM670A_HwAg1Meas/HwAg1Meas/HwAg1MeasHwAg1AutTrim/CopyRight2 ==

== system CM670A_HwAg1Meas/HwAg1Meas/HwAg1MeasHwAg1ClrTrim/CopyRight2 ==

== system CM670A_HwAg1Meas/HwAg1Meas/HwAg1MeasHwAg1ReadTrim/CopyRight2 ==

== system CM670A_HwAg1Meas/HwAg1Meas/HwAg1MeasHwAg1TrimPrfmdSts/CopyRight2 ==

== system CM670A_HwAg1Meas/HwAg1Meas/HwAg1MeasHwAg1WrTrim/CopyRight2 ==

== system CM670A_HwAg1Meas/HwAg1Meas/HwAg1MeasInit1/CopyRight2 ==

== system CM670A_HwAg1Meas/HwAg1Meas/HwAg1MeasInit1/GetRefTmr1MicroSec32bit ==
  CopyRight2 : Subsystem  Description=|  mask(Copyright Information){none=on}
      | Copyright info block.                                               
      |                                                                     
      | Place copyright information at the top of every subsystem in design.
      mask prompts: none "No parameters"
      mask help: Place copyright information at the top of every subsystem in design.
      mask Display:
      | NxtrConf = 'Nexteer Confidential';
      | 
      | sys = bdroot; %handle for the current model ("system")
      | first = get_param(sys,'Created');
      | first = first(end-3:end);  %year is last four digits
      | 
      | last = get_param(sys,'LastModifiedDate');
      | if isempty(last)
      |     last = datestr(now,'yyyy');
      | else
      |     last = last(end-3:end);
      | end
      | 
      | if strcmp(first,last)
      |     fprintf('%s -- Copyright %s Nexteer',NxtrConf,first)
      | else
      |     fprintf('%s -- %s%s- %s Nexteer',NxtrConf,char(169),first,last)
      | end
  Ground : Ground
  RefTmr : Outport
  wires:
  Ground/1 -> RefTmr/1

== system CM670A_HwAg1Meas/HwAg1Meas/HwAg1MeasInit1/GetTiSpan1MicroSec32bit ==
  RefTmr : Inport
  CopyRight2 : Subsystem  Description=|  mask(Copyright Information){none=on}
      | Copyright info block.                                               
      |                                                                     
      | Place copyright information at the top of every subsystem in design.
      mask prompts: none "No parameters"
      mask help: Place copyright information at the top of every subsystem in design.
      mask Display:
      | NxtrConf = 'Nexteer Confidential';
      | 
      | sys = bdroot; %handle for the current model ("system")
      | first = get_param(sys,'Created');
      | first = first(end-3:end);  %year is last four digits
      | 
      | last = get_param(sys,'LastModifiedDate');
      | if isempty(last)
      |     last = datestr(now,'yyyy');
      | else
      |     last = last(end-3:end);
      | end
      | 
      | if strcmp(first,last)
      |     fprintf('%s -- Copyright %s Nexteer',NxtrConf,first)
      | else
      |     fprintf('%s -- %s%s- %s Nexteer',NxtrConf,char(169),first,last)
      | end
  Ground : Ground
  Terminator : Terminator
  TiSpan : Outport
  wires:
  Ground/1 -> TiSpan/1
  RefTmr/1 -> Terminator/1

== system CM670A_HwAg1Meas/HwAg1Meas/HwAg1MeasInit1/IoHwAb_SetFctPrphlHwAg1 ==
  CopyRight2 : Subsystem  Description=|  mask(Copyright Information){none=on}
      | Copyright info block.                                               
      |                                                                     
      | Place copyright information at the top of every subsystem in design.
      mask prompts: none "No parameters"
      mask help: Place copyright information at the top of every subsystem in design.
      mask Display:
      | NxtrConf = 'Nexteer Confidential';
      | 
      | sys = bdroot; %handle for the current model ("system")
      | first = get_param(sys,'Created');
      | first = first(end-3:end);  %year is last four digits
      | 
      | last = get_param(sys,'LastModifiedDate');
      | if isempty(last)
      |     last = datestr(now,'yyyy');
      | else
      |     last = last(end-3:end);
      | end
      | 
      | if strcmp(first,last)
      |     fprintf('%s -- Copyright %s Nexteer',NxtrConf,first)
      | else
      |     fprintf('%s -- %s%s- %s Nexteer',NxtrConf,char(169),first,last)
      | end

== system CM670A_HwAg1Meas/HwAg1Meas/HwAg1MeasPer1/CopyRight2 ==

== system CM670A_HwAg1Meas/HwAg1Meas/HwAg1MeasPer1/GetRefTmr1MicroSec32bit1 ==
  CopyRight2 : Subsystem  Description=|  mask(Copyright Information){none=on}
      | Copyright info block.                                               
      |                                                                     
      | Place copyright information at the top of every subsystem in design.
      mask prompts: none "No parameters"
      mask help: Place copyright information at the top of every subsystem in design.
      mask Display:
      | NxtrConf = 'Nexteer Confidential';
      | 
      | sys = bdroot; %handle for the current model ("system")
      | first = get_param(sys,'Created');
      | first = first(end-3:end);  %year is last four digits
      | 
      | last = get_param(sys,'LastModifiedDate');
      | if isempty(last)
      |     last = datestr(now,'yyyy');
      | else
      |     last = last(end-3:end);
      | end
      | 
      | if strcmp(first,last)
      |     fprintf('%s -- Copyright %s Nexteer',NxtrConf,first)
      | else
      |     fprintf('%s -- %s%s- %s Nexteer',NxtrConf,char(169),first,last)
      | end
  Ground : Ground
  RefTmr : Outport
  wires:
  Ground/1 -> RefTmr/1

== system CM670A_HwAg1Meas/HwAg1Meas/HwAg1MeasPer1/GetTiSpan1MicroSec32bit ==
  RefTmr : Inport
  CopyRight2 : Subsystem  Description=|  mask(Copyright Information){none=on}
      | Copyright info block.                                               
      |                                                                     
      | Place copyright information at the top of every subsystem in design.
      mask prompts: none "No parameters"
      mask help: Place copyright information at the top of every subsystem in design.
      mask Display:
      | NxtrConf = 'Nexteer Confidential';
      | 
      | sys = bdroot; %handle for the current model ("system")
      | first = get_param(sys,'Created');
      | first = first(end-3:end);  %year is last four digits
      | 
      | last = get_param(sys,'LastModifiedDate');
      | if isempty(last)
      |     last = datestr(now,'yyyy');
      | else
      |     last = last(end-3:end);
      | end
      | 
      | if strcmp(first,last)
      |     fprintf('%s -- Copyright %s Nexteer',NxtrConf,first)
      | else
      |     fprintf('%s -- %s%s- %s Nexteer',NxtrConf,char(169),first,last)
      | end
  Ground : Ground
  Terminator : Terminator
  TiSpan : Outport
  wires:
  RefTmr/1 -> Terminator/1
  Ground/1 -> TiSpan/1

== system CM670A_HwAg1Meas/HwAg1Meas/HwAg1MeasPer1/IncrementCount ==
  Action Port : ActionPort  ActionType=then
  Add : Sum
  Constant : Constant  OutDataTypeStr=uint8
  CopyRight2 : Subsystem  Description=|  mask(Copyright Information){none=on}
      | Copyright info block.                                               
      |                                                                     
      | Place copyright information at the top of every subsystem in design.
      mask prompts: none "No parameters"
      mask help: Place copyright information at the top of every subsystem in design.
      mask Display:
      | NxtrConf = 'Nexteer Confidential';
      | 
      | sys = bdroot; %handle for the current model ("system")
      | first = get_param(sys,'Created');
      | first = first(end-3:end);  %year is last four digits
      | 
      | last = get_param(sys,'LastModifiedDate');
      | if isempty(last)
      |     last = datestr(now,'yyyy');
      | else
      |     last = last(end-3:end);
      | end
      | 
      | if strcmp(first,last)
      |     fprintf('%s -- Copyright %s Nexteer',NxtrConf,first)
      | else
      |     fprintf('%s -- %s%s- %s Nexteer',NxtrConf,char(169),first,last)
      | end
  Data Store Read : DataStoreRead  DataStoreName=HwAg1SnsrTrigNr
  Data Store Write : DataStoreWrite  DataStoreName=HwAg1SnsrTrigNr
  wires:
  Add/1 -> Data Store Write/1
  Data Store Read/1 -> Add/1
  Constant/1 -> Add/2

== stateflow chart CM670A_HwAg1Meas/HwAg1Meas/HwAg1MeasPer4/HwAgRead/RollCnt ==
  settings: stateMachineType=MEALY_MACHINE
  (default) -> (junction 89) : {HwAg1RollgCntr = HwAg1MeasPrevRollCnt;}
  (junction 89) -> (junction 169) [order 1] : [ (TestOk ==2) || (TestOk ==0) ]
  (junction 89) -> (junction 93) [order 2] : {
      | HwAg1RollgCntr = HwAg1RollgCntr;
      | }
  (junction 169) -> (junction 93) [order 2] : {HwAg1RollgCntr = 0;}
  (junction 169) -> (junction 93) [order 1] : [(HwAg1RollgCntr+1) <= 255]
      | {HwAg1RollgCntr = HwAg1RollgCntr + 1;}
  (junction 93) -> (junction 188)
  data: HwAg1RollgCntr output uint8; TestOk input uint8; HwAg1MeasPrevRollCnt input uint8

== stateflow chart CM670A_HwAg1Meas/HwAg1Meas/HwAg1MeasPer4/HwAgRead/If Action Subsystem/SetNtcSts/ISO Fault Debounce Design ==
  settings: stateMachineType=MEALY_MACHINE
  note: NTCSTS_PASSD           (0)
      | NTCSTS_FAILD             (1)
      | NTCSTS_PREPASSD   (2)
      | NTCSTS_PREFAILD     (3)
      |
      | SIGQLFR_NORES        (0)
      | SIGQLFR_PASSD         (1)
      | SIGQLFR_FAILD           (2)
  note: Pass Loop
  note: Fail Loop
  note: 
  (default) -> (junction 89)
  (junction 89) -> (junction 95) [order 1] : [NtcSts ==3]
  (junction 89) -> (junction 93) [order 2] : [NtcSts ==2]
  (junction 89) -> (junction 141) [order 3] : [NtcSts ==1]
      | { ErrAcc = 32767;
      | Qualifier =2;
      |  }
  (junction 89) -> (junction 141) [order 4] : [NtcSts ==0]
      | { ErrAcc = -32768;
      | Qualifier=1;
      | }
  (junction 95) -> (junction 103) [order 2]
  (junction 95) -> (junction 111) [order 1] : [ErrAcc <=0]
      | {ErrAcc = DebStep;}
  (junction 93) -> (junction 123) [order 2] : {
      | ErrAcc = ErrAcc - DebStep;
      | }
  (junction 93) -> (junction 123) [order 1] : [(ErrAcc - DebStep) <= -32768]
      | { ErrAcc = -32768;
      | Qualifier=1;
      | }
  (junction 103) -> (junction 111) [order 1] : [(ErrAcc + DebStep) <32767]
      | {ErrAcc = ErrAcc + DebStep;}
  (junction 103) -> (junction 111) [order 2] : {ErrAcc = 32767;
      | Qualifier =2;}
  (junction 123) -> (junction 141)
  (junction 111) -> (junction 141)
  (junction 141) -> (junction 159) [order 2] : {ErrAcc = 0;
      | Qualifier =0;
      | }
  (junction 141) -> (junction 159) [order 1] : [SvcClr ==0]
  data: NtcSts input uint8; Qualifier output uint8; DebStep input uint16; ErrAcc local single; SvcClr input

== stateflow chart CM670A_HwAg1Meas/HwAg1Meas/HwAg1MeasPer5/SetNtcSts/ISO Fault Debounce Design ==
  settings: stateMachineType=MEALY_MACHINE
  note: NTCSTS_PASSD           (0)
      | NTCSTS_FAILD             (1)
      | NTCSTS_PREPASSD   (2)
      | NTCSTS_PREFAILD     (3)
      |
      | SIGQLFR_NORES        (0)
      | SIGQLFR_PASSD         (1)
      | SIGQLFR_FAILD           (2)
  note: Pass Loop
  note: Fail Loop
  note: 
  (default) -> (junction 89)
  (junction 89) -> (junction 95) [order 1] : [NtcSts ==3]
  (junction 89) -> (junction 93) [order 2] : [NtcSts ==2]
  (junction 89) -> (junction 141) [order 3] : [NtcSts ==1]
      | { ErrAcc = 32767;
      | Qualifier =2;
      |  }
  (junction 89) -> (junction 141) [order 4] : [NtcSts ==0]
      | { ErrAcc = -32768;
      | Qualifier=1;
      | }
  (junction 95) -> (junction 103) [order 2]
  (junction 95) -> (junction 111) [order 1] : [ErrAcc <=0]
      | {ErrAcc = DebStep;}
  (junction 93) -> (junction 123) [order 2] : {
      | ErrAcc = ErrAcc - DebStep;
      | }
  (junction 93) -> (junction 123) [order 1] : [(ErrAcc - DebStep) <= -32768]
      | { ErrAcc = -32768;
      | Qualifier=1;
      | }
  (junction 103) -> (junction 111) [order 1] : [(ErrAcc + DebStep) <32767]
      | {ErrAcc = ErrAcc + DebStep;}
  (junction 103) -> (junction 111) [order 2] : {ErrAcc = 32767;
      | Qualifier =2;}
  (junction 123) -> (junction 141)
  (junction 111) -> (junction 141)
  (junction 141) -> (junction 159) [order 2] : {ErrAcc = 0;
      | Qualifier =0;
      | }
  (junction 141) -> (junction 159) [order 1] : [SvcClr ==0]
  data: NtcSts input uint8; Qualifier output uint8; DebStep input uint16; ErrAcc local single; SvcClr input

== system CM670A_HwAg1Meas/HwAg1Meas/HwAg1MeasPer1/ResetCount ==
  Action Port : ActionPort  ActionType=else
  Constant1 : Constant  Value=HWAG10THTOOTHTRIG_CNT_U08
      settings: AttributesFormatString=%<Value>.EngVal = 1
  CopyRight2 : Subsystem  Description=|  mask(Copyright Information){none=on}
      | Copyright info block.                                               
      |                                                                     
      | Place copyright information at the top of every subsystem in design.
      mask prompts: none "No parameters"
      mask help: Place copyright information at the top of every subsystem in design.
      mask Display:
      | NxtrConf = 'Nexteer Confidential';
      | 
      | sys = bdroot; %handle for the current model ("system")
      | first = get_param(sys,'Created');
      | first = first(end-3:end);  %year is last four digits
      | 
      | last = get_param(sys,'LastModifiedDate');
      | if isempty(last)
      |     last = datestr(now,'yyyy');
      | else
      |     last = last(end-3:end);
      | end
      | 
      | if strcmp(first,last)
      |     fprintf('%s -- Copyright %s Nexteer',NxtrConf,first)
      | else
      |     fprintf('%s -- %s%s- %s Nexteer',NxtrConf,char(169),first,last)
      | end
  Data Store Write : DataStoreWrite  DataStoreName=HwAg1SnsrTrigNr
  wires:
  Constant1/1 -> Data Store Write/1

== system CM670A_HwAg1Meas/HwAg1Meas/HwAg1MeasPer2/CopyRight2 ==

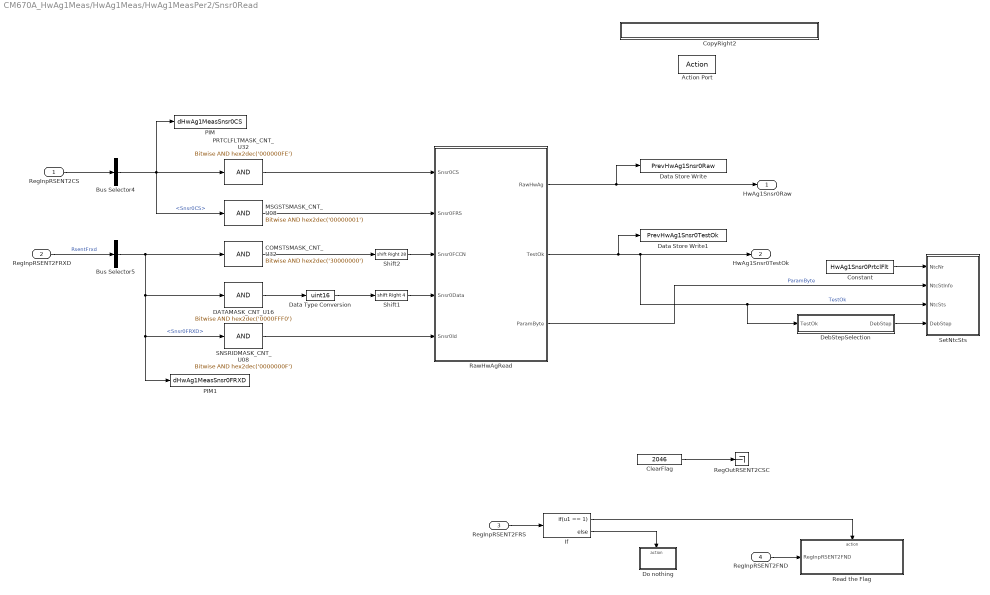
== system CM670A_HwAg1Meas/HwAg1Meas/HwAg1MeasPer2/Snsr0Read ==
  RegInpRSENT2CS : Inport
  RegInpRSENT2FRXD : Inport  Port=2
  RegInpRSENT2FRS : Inport  Port=3
  RegInpRSENT2FND : Inport  Port=4
  Action Port : ActionPort  ActionType=then
  Bus Selector4 : BusSelector  OutputSignals=Snsr0CS
  Bus Selector5 : BusSelector  OutputSignals=Snsr0FRXD
  COMSTSMASK_CNT_U32 : simulink/Logic and Bit Operations/Bitwise Operator  logicop=AND  UseBitMask=on  BitMask=hex2dec('30000000')  BitMaskRealWorld=Stored Integer
  ClearFlag : Constant  RequirementInfo={} %GIDa_43d713c2_c28c_491b_8b2b_a2f111750c85  Value=2046  OutDataTypeStr=uint16
  Constant : Constant  Value=HwAg1Snsr0PrtclFlt
  CopyRight2 : Subsystem  Description=|  mask(Copyright Information){none=on}
      | Copyright info block.                                               
      |                                                                     
      | Place copyright information at the top of every subsystem in design.
      mask prompts: none "No parameters"
      mask help: Place copyright information at the top of every subsystem in design.
      mask Display:
      | NxtrConf = 'Nexteer Confidential';
      | 
      | sys = bdroot; %handle for the current model ("system")
      | first = get_param(sys,'Created');
      | first = first(end-3:end);  %year is last four digits
      | 
      | last = get_param(sys,'LastModifiedDate');
      | if isempty(last)
      |     last = datestr(now,'yyyy');
      | else
      |     last = last(end-3:end);
      | end
      | 
      | if strcmp(first,last)
      |     fprintf('%s -- Copyright %s Nexteer',NxtrConf,first)
      | else
      |     fprintf('%s -- %s%s- %s Nexteer',NxtrConf,char(169),first,last)
      | end
  DATAMASK_CNT_U16 : simulink/Logic and Bit Operations/Bitwise Operator  logicop=AND  UseBitMask=on  BitMask=hex2dec('0000FFF0')  BitMaskRealWorld=Stored Integer
  Data Store Write : DataStoreWrite  DataStoreName=PrevHwAg1Snsr0Raw
  Data Store Write1 : DataStoreWrite  DataStoreName=PrevHwAg1Snsr0TestOk
  Data Type Conversion : DataTypeConversion  OutDataTypeStr=uint16
  DebStepSelection : Subsystem
  Do nothing : Subsystem  RequirementInfo={} %GIDa_7c28e56e_0bf6_457e_b8f1_f117d54afbe5  TreatAsAtomicUnit=on
  If : If  RequirementInfo={} %GIDa_16428bd5_cc3d_48ac_b1dc_a0997843e59c  IfExpression=u1 == 1
  MSGSTSMASK_CNT_U08 : simulink/Logic and Bit Operations/Bitwise Operator  logicop=AND  UseBitMask=on  BitMask=hex2dec('00000001')  BitMaskRealWorld=Stored Integer
  PIM : DataStoreWrite  RequirementInfo={} %GIDa_ba3ef3a3_15e1_45fd_adbd_24e50e4e1a9e  DataStoreName=dHwAg1MeasSnsr0CS
  PIM1 : DataStoreWrite  RequirementInfo={} %GIDa_d13d771c_08f2_46ee_8bc7_607b5b4cdc08  DataStoreName=dHwAg1MeasSnsr0FRXD
  PRTCLFLTMASK_CNT_U32 : simulink/Logic and Bit Operations/Bitwise Operator  logicop=AND  UseBitMask=on  BitMask=hex2dec('000000FE')  BitMaskRealWorld=Stored Integer
  RawHwAgRead : Subsystem  RequirementInfo={'linktype_rmi_doors' '0000cf44 (/ESG Group/FDD Module Requirements/EA4 Specific/CM670A_HwAg1Meas)' '#CM670A_27' 'true' 'REQ: CM670A_27' '' } %GIDa_bbc58719_dac6_409b_b71b_1d93741cf29f
  Read the Flag : Subsystem  RequirementInfo={} %GIDa_2fc9c043_d528_4c42_b878_d48a787d3c50  TreatAsAtomicUnit=on
  RegOutRSENT2CSC : Terminator
  SNSRIDMASK_CNT_U08 : simulink/Logic and Bit Operations/Bitwise Operator  logicop=AND  UseBitMask=on  BitMask=hex2dec('0000000F')  BitMaskRealWorld=Stored Integer
  SetNtcSts : Subsystem  RequirementInfo={'linktype_rmi_doors' '0000cf44 (/ESG Group/FDD Module Requirements/EA4 Specific/CM670A_HwAg1Meas)' '#CM670A_38' 'true' 'REQ: CM670A_38' '' } %GIDa_4b9b3dda_1259_42b5_920e_682aedf8ad34
  Shift1 : ArithShift  BitShiftNumber=4  BitShiftDirection=Right
  Shift2 : ArithShift  BitShiftNumber=28  BitShiftDirection=Right
  HwAg1Snsr0Raw : Outport
  HwAg1Snsr0TestOk : Outport  Port=2
  wires:
  RawHwAgRead/1(RawHwAg) -> Data Store Write/1, HwAg1Snsr0Raw/1
  RawHwAgRead/2(TestOk) -> Data Store Write1/1, DebStepSelection/1(TestOk), SetNtcSts/3(NtcSts), HwAg1Snsr0TestOk/1  "TestOk"
  RawHwAgRead/3(ParamByte) -> SetNtcSts/2(NtcStInfo)  "ParamByte"
  DebStepSelection/1(DebStep) -> SetNtcSts/4(DebStep)
  Constant/1 -> SetNtcSts/1(NtcNr)
  PRTCLFLTMASK_CNT_U32/1 -> RawHwAgRead/1(Snsr0CS)
  MSGSTSMASK_CNT_U08/1 -> RawHwAgRead/2(Snsr0FRS)
  COMSTSMASK_CNT_U32/1 -> Shift2/1
  RegInpRSENT2FRXD/1 -> Bus Selector5/1  "RsentFrxd"
  DATAMASK_CNT_U16/1 -> Data Type Conversion/1
  SNSRIDMASK_CNT_U08/1 -> RawHwAgRead/5(Snsr0Id)
  Shift1/1 -> RawHwAgRead/4(Snsr0Data)
  Shift2/1 -> RawHwAgRead/3(Snsr0FCCN)
  Bus Selector4/1 -> PIM/1, MSGSTSMASK_CNT_U08/1, PRTCLFLTMASK_CNT_U32/1  "<Snsr0CS>"
  Bus Selector5/1 -> PIM1/1, SNSRIDMASK_CNT_U08/1, DATAMASK_CNT_U16/1, COMSTSMASK_CNT_U32/1  "<Snsr0FRXD>"
  Data Type Conversion/1 -> Shift1/1
  RegInpRSENT2CS/1 -> Bus Selector4/1
  ClearFlag/1 -> RegOutRSENT2CSC/1
  RegInpRSENT2FRS/1 -> If/1
  If/1 -> Read the Flag/Action
  If/2 -> Do nothing/Action
  RegInpRSENT2FND/1 -> Read the Flag/1(RegInpRSENT2FND)

== system CM670A_HwAg1Meas/HwAg1Meas/HwAg1MeasPer2/Snsr0Read1 ==
  Action Port : ActionPort  ActionType=else
  CopyRight2 : Subsystem  Description=|  mask(Copyright Information){none=on}
      | Copyright info block.                                               
      |                                                                     
      | Place copyright information at the top of every subsystem in design.
      mask prompts: none "No parameters"
      mask help: Place copyright information at the top of every subsystem in design.
      mask Display:
      | NxtrConf = 'Nexteer Confidential';
      | 
      | sys = bdroot; %handle for the current model ("system")
      | first = get_param(sys,'Created');
      | first = first(end-3:end);  %year is last four digits
      | 
      | last = get_param(sys,'LastModifiedDate');
      | if isempty(last)
      |     last = datestr(now,'yyyy');
      | else
      |     last = last(end-3:end);
      | end
      | 
      | if strcmp(first,last)
      |     fprintf('%s -- Copyright %s Nexteer',NxtrConf,first)
      | else
      |     fprintf('%s -- %s%s- %s Nexteer',NxtrConf,char(169),first,last)
      | end
  Data Store Read : DataStoreRead  DataStoreName=PrevHwAg1Snsr0Raw
  Data Store Read1 : DataStoreRead  DataStoreName=PrevHwAg1Snsr0TestOk
  HwAg1Snsr0Raw : Outport
  HwAg1Snsr0TestOk : Outport  Port=2
  wires:
  Data Store Read1/1 -> HwAg1Snsr0TestOk/1
  Data Store Read/1 -> HwAg1Snsr0Raw/1

== system CM670A_HwAg1Meas/HwAg1Meas/HwAg1MeasPer3/CopyRight2 ==

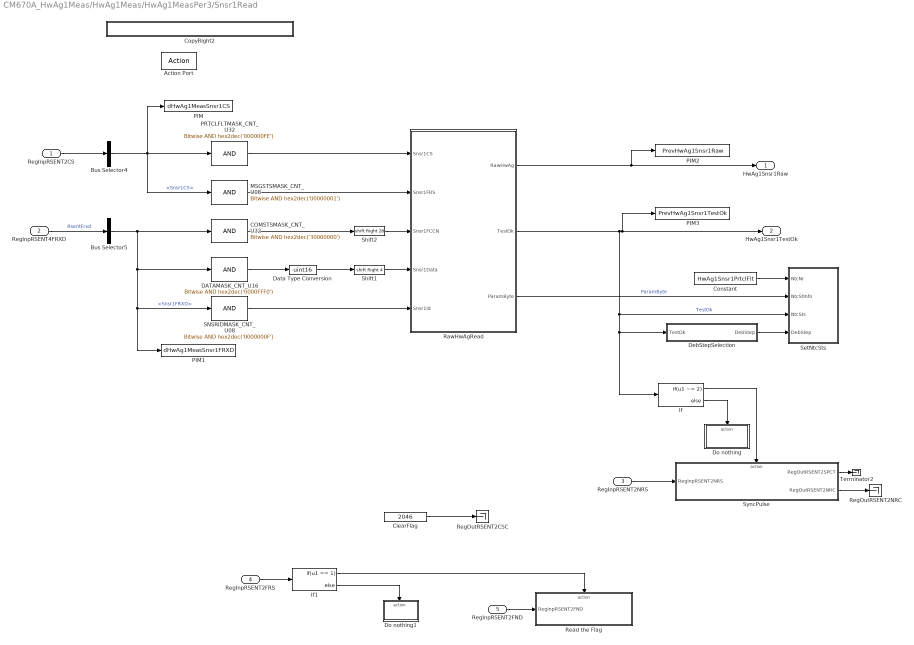
== system CM670A_HwAg1Meas/HwAg1Meas/HwAg1MeasPer3/Snsr1Read ==
  RegInpRSENT2CS : Inport
  RegInpRSENT4FRXD : Inport  Port=2
  RegInpRSENT2NRS : Inport  Port=3
  RegInpRSENT2FRS : Inport  Port=4
  RegInpRSENT2FND : Inport  Port=5
  Action Port : ActionPort  ActionType=then
  Bus Selector4 : BusSelector  OutputSignals=Snsr1CS
  Bus Selector5 : BusSelector  OutputSignals=Snsr1FRXD
  COMSTSMASK_CNT_U32 : simulink/Logic and Bit Operations/Bitwise Operator  logicop=AND  UseBitMask=on  BitMask=hex2dec('30000000')  BitMaskRealWorld=Stored Integer
  ClearFlag : Constant  RequirementInfo={} %GIDa_d535d42f_ec14_4cf2_97f7_8ebd19e6feea  Value=2046  OutDataTypeStr=uint16
  Constant : Constant  Value=HwAg1Snsr1PrtclFlt
  CopyRight2 : Subsystem  Description=|  mask(Copyright Information){none=on}
      | Copyright info block.                                               
      |                                                                     
      | Place copyright information at the top of every subsystem in design.
      mask prompts: none "No parameters"
      mask help: Place copyright information at the top of every subsystem in design.
      mask Display:
      | NxtrConf = 'Nexteer Confidential';
      | 
      | sys = bdroot; %handle for the current model ("system")
      | first = get_param(sys,'Created');
      | first = first(end-3:end);  %year is last four digits
      | 
      | last = get_param(sys,'LastModifiedDate');
      | if isempty(last)
      |     last = datestr(now,'yyyy');
      | else
      |     last = last(end-3:end);
      | end
      | 
      | if strcmp(first,last)
      |     fprintf('%s -- Copyright %s Nexteer',NxtrConf,first)
      | else
      |     fprintf('%s -- %s%s- %s Nexteer',NxtrConf,char(169),first,last)
      | end
  DATAMASK_CNT_U16 : simulink/Logic and Bit Operations/Bitwise Operator  logicop=AND  UseBitMask=on  BitMask=hex2dec('0000FFF0')  BitMaskRealWorld=Stored Integer
  Data Type Conversion : DataTypeConversion  OutDataTypeStr=uint16
  DebStepSelection : Subsystem
  Do nothing : Subsystem  RequirementInfo={} %GIDa_fbce4302_0ab7_4bfe_bcff_1a100a372b73  TreatAsAtomicUnit=on
  Do nothing1 : Subsystem  RequirementInfo={} %GIDa_a153506d_e67e_4c18_8ee2_923bcd11a2d2  TreatAsAtomicUnit=on
  If : If  RequirementInfo={} %GIDa_b00b24bd_2a6f_4e26_a22a_ba6cbf670068  IfExpression=u1 ~= 2
  If1 : If  RequirementInfo={} %GIDa_381a7916_6331_404f_af2d_d019ea7e60c7  IfExpression=u1 == 1
  MSGSTSMASK_CNT_U08 : simulink/Logic and Bit Operations/Bitwise Operator  logicop=AND  UseBitMask=on  BitMask=hex2dec('00000001')  BitMaskRealWorld=Stored Integer
  PIM : DataStoreWrite  RequirementInfo={} %GIDa_d1d3e16b_3567_4159_a1ee_fc50af325c45  DataStoreName=dHwAg1MeasSnsr1CS
  PIM1 : DataStoreWrite  RequirementInfo={} %GIDa_109d8734_7cde_49f2_afa9_05b41adc6c19  DataStoreName=dHwAg1MeasSnsr1FRXD
  PIM2 : DataStoreWrite  RequirementInfo={} %GIDa_e4da1725_a102_443f_844c_8a9f8cdb572d  DataStoreName=PrevHwAg1Snsr1Raw
  PIM3 : DataStoreWrite  RequirementInfo={} %GIDa_93839c12_c479_4722_b3a2_6d7a3605f0ae  DataStoreName=PrevHwAg1Snsr1TestOk
  PRTCLFLTMASK_CNT_U32 : simulink/Logic and Bit Operations/Bitwise Operator  logicop=AND  UseBitMask=on  BitMask=hex2dec('000000FE')  BitMaskRealWorld=Stored Integer
  RawHwAgRead : Subsystem  RequirementInfo={'linktype_rmi_doors' '0000cf44 (/ESG Group/FDD Module Requirements/EA4 Specific/CM670A_HwAg1Meas)' '#CM670A_27' 'true' 'REQ: CM670A_27' '' } %GIDa_4fff3f05_9e59_4702_98bd_3cdadb9e3d81
  Read the Flag : Subsystem  RequirementInfo={} %GIDa_e753e0b4_7435_4b1a_be97_79dffab10527  TreatAsAtomicUnit=on
  RegOutRSENT2CSC : Terminator
  RegOutRSENT2NRC : Terminator
  SNSRIDMASK_CNT_U08 : simulink/Logic and Bit Operations/Bitwise Operator  logicop=AND  UseBitMask=on  BitMask=hex2dec('0000000F')  BitMaskRealWorld=Stored Integer
  SetNtcSts : Subsystem  RequirementInfo={'linktype_rmi_doors' '0000cf44 (/ESG Group/FDD Module Requirements/EA4 Specific/CM670A_HwAg1Meas)' '#CM670A_58' 'true' 'REQ: CM670A_58' '' } %GIDa_95bfa482_64f2_4b7f_bc5c_d3f205b75ab8
  Shift1 : ArithShift  BitShiftNumber=4  BitShiftDirection=Right
  Shift2 : ArithShift  BitShiftNumber=28  BitShiftDirection=Right
  SyncPulse : Subsystem  RequirementInfo={} %GIDa_245be4ad_5058_43f8_b993_7f8673538233  TreatAsAtomicUnit=on
  Terminator2 : Terminator
  HwAg1Snsr1Raw : Outport
  HwAg1Snsr1TestOk : Outport  Port=2
  wires:
  RawHwAgRead/3(ParamByte) -> SetNtcSts/2(NtcStInfo)  "ParamByte"
  DebStepSelection/1(DebStep) -> SetNtcSts/4(DebStep)
  Constant/1 -> SetNtcSts/1(NtcNr)
  RawHwAgRead/1(RawHwAg) -> PIM2/1, HwAg1Snsr1Raw/1
  PRTCLFLTMASK_CNT_U32/1 -> RawHwAgRead/1(Snsr1CS)
  MSGSTSMASK_CNT_U08/1 -> RawHwAgRead/2(Snsr1FRS)
  COMSTSMASK_CNT_U32/1 -> Shift2/1
  RegInpRSENT4FRXD/1 -> Bus Selector5/1  "RsentFrxd"
  DATAMASK_CNT_U16/1 -> Data Type Conversion/1
  SNSRIDMASK_CNT_U08/1 -> RawHwAgRead/5(Snsr1Id)
  Shift1/1 -> RawHwAgRead/4(Snsr1Data)
  Shift2/1 -> RawHwAgRead/3(Snsr1FCCN)
  Bus Selector4/1 -> PIM/1, MSGSTSMASK_CNT_U08/1, PRTCLFLTMASK_CNT_U32/1  "<Snsr1CS>"
  Bus Selector5/1 -> PIM1/1, SNSRIDMASK_CNT_U08/1, DATAMASK_CNT_U16/1, COMSTSMASK_CNT_U32/1  "<Snsr1FRXD>"
  Data Type Conversion/1 -> Shift1/1
  RegInpRSENT2CS/1 -> Bus Selector4/1
  RawHwAgRead/2(TestOk) -> PIM3/1, HwAg1Snsr1TestOk/1, If/1, DebStepSelection/1(TestOk), SetNtcSts/3(NtcSts)  "TestOk"
  If/1 -> SyncPulse/Action
  If/2 -> Do nothing/Action
  SyncPulse/1(RegOutRSENT2SPCT) -> Terminator2/1
  SyncPulse/2(RegOutRSENT2NRC) -> RegOutRSENT2NRC/1
  RegInpRSENT2NRS/1 -> SyncPulse/1(RegInpRSENT2NRS)
  ClearFlag/1 -> RegOutRSENT2CSC/1
  RegInpRSENT2FRS/1 -> If1/1
  If1/1 -> Read the Flag/Action
  If1/2 -> Do nothing1/Action
  RegInpRSENT2FND/1 -> Read the Flag/1(RegInpRSENT2FND)

== system CM670A_HwAg1Meas/HwAg1Meas/HwAg1MeasPer3/Snsr1Read1 ==
  Action Port : ActionPort  ActionType=else
  CopyRight2 : Subsystem  Description=|  mask(Copyright Information){none=on}
      | Copyright info block.                                               
      |                                                                     
      | Place copyright information at the top of every subsystem in design.
      mask prompts: none "No parameters"
      mask help: Place copyright information at the top of every subsystem in design.
      mask Display:
      | NxtrConf = 'Nexteer Confidential';
      | 
      | sys = bdroot; %handle for the current model ("system")
      | first = get_param(sys,'Created');
      | first = first(end-3:end);  %year is last four digits
      | 
      | last = get_param(sys,'LastModifiedDate');
      | if isempty(last)
      |     last = datestr(now,'yyyy');
      | else
      |     last = last(end-3:end);
      | end
      | 
      | if strcmp(first,last)
      |     fprintf('%s -- Copyright %s Nexteer',NxtrConf,first)
      | else
      |     fprintf('%s -- %s%s- %s Nexteer',NxtrConf,char(169),first,last)
      | end
  Data Store Read : DataStoreRead  DataStoreName=PrevHwAg1Snsr1Raw
  Data Store Read1 : DataStoreRead  DataStoreName=PrevHwAg1Snsr1TestOk
  HwAg1Snsr1Raw : Outport
  HwAg1Snsr1TestOk : Outport  Port=2
  wires:
  Data Store Read1/1 -> HwAg1Snsr1TestOk/1
  Data Store Read/1 -> HwAg1Snsr1Raw/1

== system CM670A_HwAg1Meas/HwAg1Meas/HwAg1MeasPer4/CopyRight2 ==

== system CM670A_HwAg1Meas/HwAg1Meas/HwAg1MeasPer4/HwAgPrevRead ==
  Action Port : ActionPort  ActionType=else
  CopyRight2 : Subsystem  Description=|  mask(Copyright Information){none=on}
      | Copyright info block.                                               
      |                                                                     
      | Place copyright information at the top of every subsystem in design.
      mask prompts: none "No parameters"
      mask help: Place copyright information at the top of every subsystem in design.
      mask Display:
      | NxtrConf = 'Nexteer Confidential';
      | 
      | sys = bdroot; %handle for the current model ("system")
      | first = get_param(sys,'Created');
      | first = first(end-3:end);  %year is last four digits
      | 
      | last = get_param(sys,'LastModifiedDate');
      | if isempty(last)
      |     last = datestr(now,'yyyy');
      | else
      |     last = last(end-3:end);
      | end
      | 
      | if strcmp(first,last)
      |     fprintf('%s -- Copyright %s Nexteer',NxtrConf,first)
      | else
      |     fprintf('%s -- %s%s- %s Nexteer',NxtrConf,char(169),first,last)
      | end
  Data Store Read : DataStoreRead  DataStoreName=PrevHwAg1
  Data Store Read1 : DataStoreRead  DataStoreName=HwAg1PrevRollCnt
  Data Store Read2 : DataStoreRead  DataStoreName=PrevHwAg1Qlfr
  HwAg1 : Outport  RequirementInfo={} %GIDa_ae625f63_8634_4a7c_8609_d6dc16944a76
  HwAg1Qlfr : Outport  RequirementInfo={'linktype_rmi_doors' '0000cf45 (/ESG Group/FDD Module Requirements/EA4 Specific/CM690A_HwAg0Meas)' '#CM690A_30' 'true' 'REQ: CM690A_30' '' } %GIDa_ffe70d9f_97b7_4f4a_ae14_12dd391618c7  Port=2
  HwAg1RollgCntr : Outport  RequirementInfo={'linktype_rmi_doors' '0000cf45 (/ESG Group/FDD Module Requirements/EA4 Specific/CM690A_HwAg0Meas)' '#CM690A_31' 'true' 'REQ: CM690A_31' '' } %GIDa_9f9e5fcb_57f8_4fca_8cba_abc1fe894640  Port=3
  wires:
  Data Store Read2/1 -> HwAg1Qlfr/1
  Data Store Read1/1 -> HwAg1RollgCntr/1
  Data Store Read/1 -> HwAg1/1
